simulink model "wall_plumbing_V2"  (R2017b)
settings: Solver=VariableStepAuto  StartTime=0.0  StopTime=tf  RelTol=1e-3  AbsTol=1e-3  EnableMultiTasking=on
values from neighbouring files (symbols this model uses):
  cistern_diam = 100    [plumbing_variables.m]
  cistern_inlet_diam = 2    [plumbing_variables.m]
  cistern_outlet_diam = 2    [plumbing_variables.m]
  swh_inlet_diam = 2    [plumbing_variables.m]
  swh_outlet_diam = 2    [plumbing_variables.m]
undefined symbols (not defined in the file or in its folder): sigbuilder_block
libraries: fl_lib x62, nesl_utility x44, sh_lib x11, simulink x5, SimscapeFluids_lib x4, powerlib_meascontrol x2
(part 2 of 2)

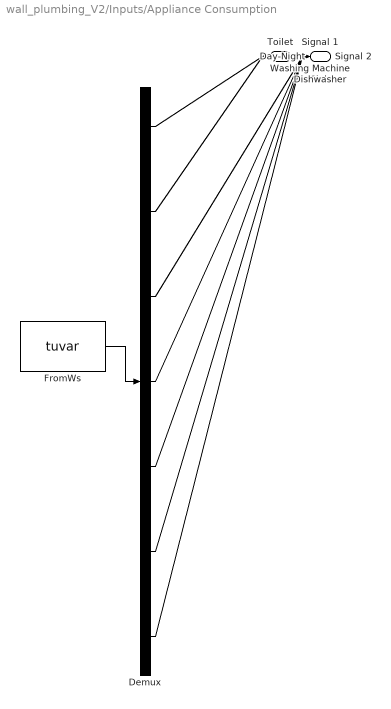
== system wall_plumbing_V2/Inputs/Appliance Consumption ==
  Demux : Demux  Tag=STV Demux  Outputs=7
  FromWs : FromWorkspace  Tag=STV FromWs  VariableName=tuvar  SampleTime=0
      SigBuilderData=|
      | common.afterFinalStr = 'Extrapolate'
      | common.sampleTime = 0
      | dataSet.timeRange = [0 604800]
      | dataSet.name = 'Group 1'
      | sbobj.Groups.Name = 'Group 1'
      | sbobj.Groups.Signals(1).Name = 'Toilet'
      | sbobj.Groups.Signals(1).XData = [0 30 30 3600 3600 3630 3630 7200 7200 7230 7230 10800 ... (672 elements, 1x672)]
      | sbobj.Groups.Signals(1).YData = [2 2 0 0 2 2 0 0 2 2 0 0 2 2 0 0 2 2 0 0 2 2 0 0 2 2 0 0 2 2 0 0 2 2 0 0 2 2 0 0 2 2 0 0 2 2 0 0 2 2 0 0 2 2 0 0 2 2 0 0 2 2 0 0 2 2 0 0 2 2 0 0 2 2 0 0 2 2 0 0 2 2 0 0 2 2 0 0 2 2 0 0 2 2 0 0 2 2 0 0 2 2 0 0 2 2 0 0 2 2 0 0 2 2 0 0 2 2 0 0 2 2 0 0 2 2 0 0 2 2 0 0 2 2 0 0 2 2 0 0 2 2 0 0 2 2 0 0 2 2 0 0 2 2 0 0 2 2 0 0 2 2 0 0 2 2 0 0 2 2 0 0 2 2 0 0 2 2 0 0 2 2 0 0 2 2 0 0 2 2 0 0 2 2 0 0 2 2 0 0 2 2 0 0 2 2 0 0 2 2 0 0 2 2 0 0 2 2 0 0 2 2 0 0 2 2 0 0 2 2 0 0 2 2 0 0 2 2 0 0 2 2 0 0 2 2 0 0 2 2 0 0 2 2 0 0 2 2 0 0 2 2 0 0 2 2 0 0 2 2 0 0 2 2 0 0 2 2 0 0 2 2 0 0 2 2 0 0 2 2 0 0 2 2 0 0 2 2 0 0 2 2 0 0 2 2 0 0 2 2 0 0 2 2 0 0 2 2 0 0 2 2 0 0 2 2 0 0 2 2 0 0 2 2 0 0 2 2 0 0 2 2 0 0 2 2 0 0 2 2 0 0 2 2 0 0 2 2 0 0 2 2 0 0 2 2 0 0 2 2 0 0 2 2 0 0 2 2 0 0 2 2 0 0 2 2 0 0 2 2 0 0 2 2 0 0 2 2 0 0 2 2 0 0 2 2 0 0 2 2 0 0 2 2 0 0 2 2 0 0 2 2 0 0 2 2 0 0 2 2 0 0 2 2 0 0 2 2 0 0 2 2 0 0 2 2 0 0 2 2 0 0 2 2 0 0 2 2 0 0 2 2 0 0 2 2 0 0 2 2 0 0 2 2 0 0 2 2 0 0 2 2 0 0 2 2 0 0 2 2 0 0 2 2 0 0 2 2 0 0 2 2 0 0 2 2 0 0 2 2 0 0 2 2 0 0 2 2 0 0 2 2 0 0 2 2 0 0 2 2 0 0 2 2 0 0 2 2 0 0 2 2 0 0 2 2 0 0 2 2 0 0 2 2 0 0 2 2 0 0 2 2 0 0 2 2 0 0 2 2 0 0 2 2 0 0 2 2 0 0 2 2 0 0 2 2 0 0 2 2 0 0 2 2 0 0 2 2 0 0 2 2 0 0 2 2 0 0 2 2 0 0 2 2 0 0 2 2 0 0 2 2 0 0 2 2 0 0 2 2 0 0 2 2 0 0 2 2 0 0 2 2 0 0 2 2 0 0 2 2 0 0 2 2 0 0 2 2 0 0 2 2 0 0 2 2 0 0 2 2 0 0]
      | sbobj.Groups.Signals(2).Name = 'Washing Machine'
      | sbobj.Groups.Signals(2).XData = [0 1050 1050 302400 302400 303450 303450 604800]
      | sbobj.Groups.Signals(2).YData = [0.9 0.9 0 0 2 2 0 0]
      | sbobj.Groups.Signals(3).Name = 'Signal 1'
      | sbobj.Groups.Signals(3).XData = [0 600 600 900 900 1500 1500 1800 1800 2400 2400 2700 ... (2688 elements, 1x2688)]
      | sbobj.Groups.Signals(3).YData = [2 2 0 0 2 2 0 0 2 2 0 0 ... (2688 elements, 1x2688)]
      | sbobj.Groups.Signals(4).Name = 'Signal 2'
      | sbobj.Groups.Signals(4).XData = [0 3600 3600 86400 86400 90000 90000 172800 172800 176400 176400 259200 259200 262800 262800 345600 345600 349200 349200 432000 432000 435600 435600 518400 518400 522000 522000 604800]
      | sbobj.Groups.Signals(4).YData = [1 1 0 0 1 1 0 0 1 1 0 0 1 1 0 0 1 1 0 0 1 1 0 0 1 1 0 0]
      | sbobj.Groups.Signals(5).Name = 'Sink'
      | sbobj.Groups.Signals(5).XData = [0 30 30 1200 1200 1230 1230 2400 2400 2430 2430 3600 ... (2016 elements, 1x2016)]
      | sbobj.Groups.Signals(5).YData = [2 2 0 0 2 2 0 0 2 2 0 0 ... (2016 elements, 1x2016)]
      | sbobj.Groups.Signals(6).Name = 'Dishwasher'
      | sbobj.Groups.Signals(6).XData = [0 840 840 201600 201600 202440 202440 403200 403200 404040 404040 604800]
      | sbobj.Groups.Signals(6).YData = [2 2 0 0 2 2 0 0 2 2 0 0]
      | sbobj.Groups.Signals(7).Name = 'Day-Night'
      | sbobj.Groups.Signals(7).XData = [0 57600 57600 86400 86400 144000 144000 172800 172800 230400 230400 259200 259200 316800 316800 345600 345600 403200 403200 432000 432000 489600 489600 518400 518400 576000 576000 604800]
      | sbobj.Groups.Signals(7).YData = [1 1 0 0 1 1 0 0 1 1 0 0 1 1 0 0 1 1 0 0 1 1 0 0 1 1 0 0]
      | sbobj.Groups.TimeRange = [0 604800]
  Toilet : Outport  Tag=STV Outport
  Washing Machine : Outport  Tag=STV Outport  Port=2
  Signal 1 : Outport  Tag=STV Outport  Port=3
  Signal 2 : Outport  Tag=STV Outport  Port=4
  Sink : Outport  Tag=STV Outport  Port=5
  Dishwasher : Outport  Tag=STV Outport  Port=6
  Day-Night : Outport  Tag=STV Outport  Port=7
  wires:
  FromWs/1 -> Demux/1
  Demux/1 -> Toilet/1
  Demux/2 -> Washing Machine/1
  Demux/3 -> Signal 1/1
  Demux/4 -> Signal 2/1
  Demux/5 -> Sink/1
  Demux/6 -> Dishwasher/1
  Demux/7 -> Day-Night/1

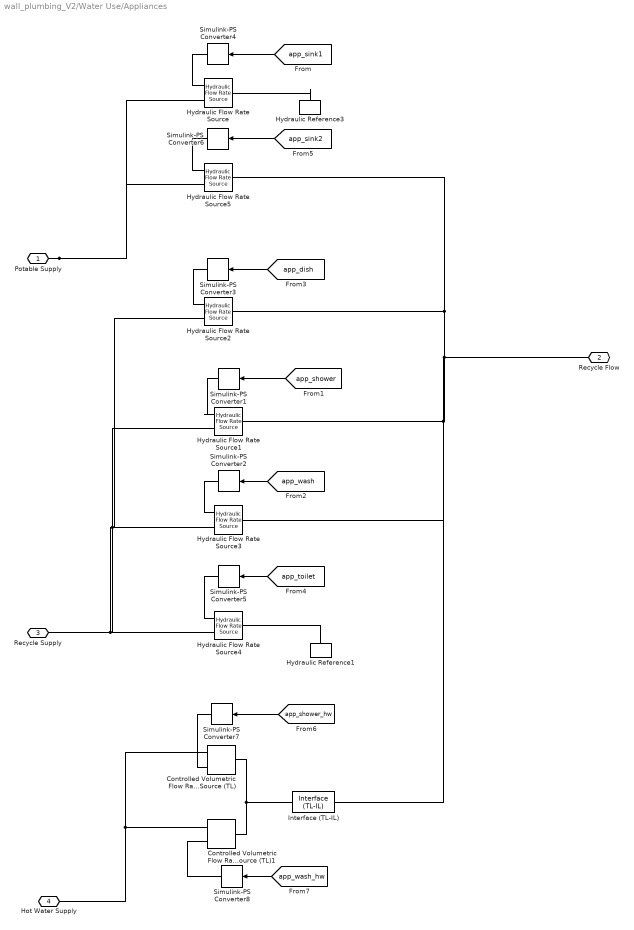
== system wall_plumbing_V2/Water Use/Appliances ==
  Controlled Volumetric Flow Rate Source (TL) : fl_lib/Thermal Liquid/Sources/Controlled Volumetric Flow Rate Source (TL)  area=pi*.25^2 in^2  length=0.1 m  mdot_A_specify=off  mdot_A_priority=None  mdot_A=1 kg/s  mdot_A_nominal_specify=off  mdot_A_nominal_unit=kg/s  mdot_A_nominal_value=1
      settings: SourceProductName=Simscape  SourceProductBaseCode=SS
  Controlled Volumetric Flow Rate Source (TL)1 : fl_lib/Thermal Liquid/Sources/Controlled Volumetric Flow Rate Source (TL)  area=pi*.25^2 in^2  length=0.1 m  mdot_A_specify=off  mdot_A_priority=None  mdot_A=1 kg/s  mdot_A_nominal_specify=off  mdot_A_nominal_unit=kg/s  mdot_A_nominal_value=1
      settings: SourceProductName=Simscape  SourceProductBaseCode=SS
  Hydraulic Flow Rate Source{,1..5} (6 alike) : fl_lib/Hydraulic/Hydraulic Sources/Hydraulic Flow Rate Source
      settings: SourceProductName=Simscape  SourceProductBaseCode=SS
  Hydraulic Reference1 : fl_lib/Hydraulic/Hydraulic Elements/Hydraulic Reference
      settings: SourceProductName=Simscape
  Hydraulic Reference3 : fl_lib/Hydraulic/Hydraulic Elements/Hydraulic Reference
      settings: SourceProductName=Simscape
  Interface (TL-IL) : SimscapeFluids_lib/Fluid Network Interfaces/Interface (TL-IL)  T_B=293.15 K  area=0.01 m^2
      settings: SourceProductName=Simscape Fluids  SourceProductBaseCode=SH
  Simulink-PS Converter{1..8} (8 alike) : nesl_utility/Simulink-PS Converter  PhysicalDomain=network_engine_domain  SubClassName=ps_input  LeftPortType=input  RightPortType=output  PseudoPeriodic=off  Frequencies=[]  NoiseDistribution=none  NoiseParameters=[]  Unit=gal/min  AffineConversion=off  FilteringAndDerivatives=zero  SimscapeFilterOrder=1  InputFilterTimeConstant=0.001  UdotUserProvided=1
  Potable Supply : PMIOPort  Port=1  Side=Left
  Recycle Flow : PMIOPort  Port=2  Side=Right
  Recycle Supply : PMIOPort  Port=3  Side=Left
  Hot Water Supply : PMIOPort  Port=4  Side=Left
  wires:
  [app_sink1] -> Simulink-PS Converter4/1
  [app_wash] -> Simulink-PS Converter2/1
  [app_dish] -> Simulink-PS Converter3/1
  [app_toilet] -> Simulink-PS Converter5/1
  [app_shower] -> Simulink-PS Converter1/1
  [app_sink2] -> Simulink-PS Converter6/1
  [app_shower_hw] -> Simulink-PS Converter7/1
  [app_wash_hw] -> Simulink-PS Converter8/1
  connections:
  Potable Supply/RConn1 -- Hydraulic Flow Rate Source5/RConn2 -- Hydraulic Flow Rate Source/RConn2
  Recycle Supply/RConn1 -- Hydraulic Flow Rate Source2/RConn2 -- Hydraulic Flow Rate Source1/RConn2 -- Hydraulic Flow Rate Source3/RConn2 -- Hydraulic Flow Rate Source4/RConn2
  Hydraulic Flow Rate Source/RConn1 -- Simulink-PS Converter4/RConn1
  Hydraulic Flow Rate Source3/RConn1 -- Simulink-PS Converter2/RConn1
  Hydraulic Flow Rate Source2/RConn1 -- Simulink-PS Converter3/RConn1
  Hydraulic Flow Rate Source4/RConn1 -- Simulink-PS Converter5/RConn1
  Hydraulic Flow Rate Source5/LConn1 -- Interface (TL-IL)/RConn1 -- Hydraulic Flow Rate Source3/LConn1 -- Hydraulic Flow Rate Source1/LConn1 -- Recycle Flow/RConn1 -- Hydraulic Flow Rate Source2/LConn1
  Hydraulic Flow Rate Source4/LConn1 -- Hydraulic Reference1/LConn1
  Hydraulic Flow Rate Source1/RConn1 -- Simulink-PS Converter1/RConn1
  Hydraulic Flow Rate Source5/RConn1 -- Simulink-PS Converter6/RConn1
  Hydraulic Reference3/LConn1 -- Hydraulic Flow Rate Source/LConn1
  Hot Water Supply/RConn1 -- Controlled Volumetric Flow Rate Source (TL)1/LConn1 -- Controlled Volumetric Flow Rate Source (TL)/LConn1
  Simulink-PS Converter7/RConn1 -- Controlled Volumetric Flow Rate Source (TL)/LConn2
  Simulink-PS Converter8/RConn1 -- Controlled Volumetric Flow Rate Source (TL)1/LConn2
  Controlled Volumetric Flow Rate Source (TL)1/RConn1 -- Interface (TL-IL)/LConn1 -- Controlled Volumetric Flow Rate Source (TL)/RConn1
